simulink model "Practica4simulink"  (R2024a)
settings: Solver=VariableStepAuto  StartTime=0.0  StopTime=10.0  RelTol=1e-3
settings Model: Creator=52331  LastModifiedBy=52331

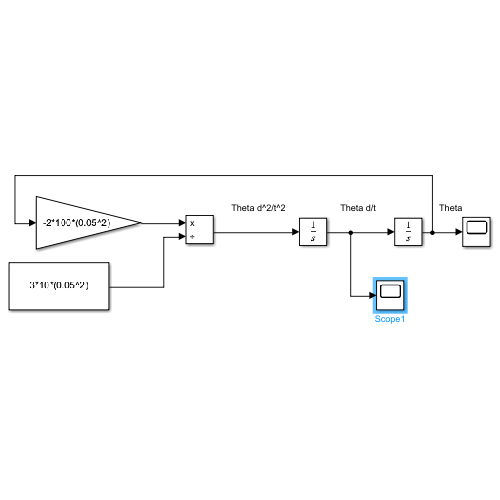
[thumbnail: Simulink's stored preview of the top-level diagram]
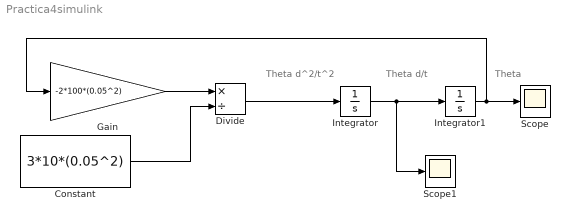
== system Practica4simulink ==
  note: Theta d^2/t^2
  note: Theta d/t
  note: Theta
  Constant : Constant  Value=3*10*(0.05^2)
  Divide : Product  Inputs=*/
  Gain : Gain  Gain=-2*100*(0.05^2)
  Integrator : Integrator  InitialCondition=2
  Integrator1 : Integrator
  Scope : Scope
  Scope1 : Scope
  wires:
  Integrator/1 -> Scope1/1, Integrator1/1
  Divide/1 -> Integrator/1
  Gain/1 -> Divide/1
  Integrator1/1 -> Scope/1, Gain/1
  Constant/1 -> Divide/2
